simulink model "LaneMerge"  (Simulink 8.2)
settings: Solver=ode1  StartTime=0.0  StopTime=Inf  FixedStep=0.001  RelTol=1e-3
PostLoadFcn:
  | , if any(exist('dsrtsu_mdlpostloadfcn', 'file') == [2, 3, 6]), try dsrtsu_mdlpostloadfcn('Execute', bdroot); catch fprintf('Error in PostLoadFcn (dsrtsu_mdlpostloadfcn) for model "%s":\n %s\n', bdroot, lasterr); end, end,
undefined symbols (not defined in the file): AccelCommandMode, command_mode, max_accel_m_s2, MergeStateEnum, override_enabled, speed_command_m_s, VehicleRoleEnum, wrench_effort_command
libraries: simulink x19, merge_activation_lib x5, dsrc_util_lib x4, dsrc_transmitter x3, carma_platform x3, srx_platform x3, merge_control_lib x2, gap_controller_lib x2, rtitttasklib x2, command_handler_lib x1, vehicle_role_lib x1, simulink_utils_lib x1
settings Model: DSRTSU_INTERNAL_RTI_VER=450  DSRTSU_INTERNAL_RTI_TYPE=rti1401  DSRTSU_INTERNAL_RTIFPGA=40  Creator=rushk1  LastModifiedBy=rushk1  BufferReuse=off
settings DataIOCC: SignalLoggingSaveFormat=Dataset
settings OptimizationCC: BlockReduction=off  OptimizeBlockIOStorage=off  BufferReuse=off  ExpressionFolding=off  ExpressionDepthLimit=128  LocalBlockOutputs=off
settings DebuggingCC: FcnCallInpInsideContextMsg=EnableAllAsError  StateNameClashWarn=none
settings HardwareCC: ProdIntDivRoundTo=Zero  ProdEndianess=BigEndian  ProdHWDeviceType=Generic->Custom  TargetHWDeviceType=Generic->Custom
settings RTWCC: SystemTargetFile=rti1401.tlc  MakeCommand=make_rti  TemplateMakefile=rti1401.tmf  Description=dSPACE DS1401 Hardware Platform  ProcessScript=rti1401_make_rtw_hook  CustomSource=command_accel_encode.c
settings STFCustomTargetCC: CodeReplacementLibrary=ANSI_C  ParMdlRefBuildCompliant=on  GeneratePreprocessorConditionals=Disable all  SystemTargetFile=rti1401.tlc
settings GRTTargetCC: CompOptLevelCompliant=off  ConcurrentExecutionCompliant=off  MatFileLogging=off  ExtModeMexFile=noextcomm
settings CustomProperty: DataType=RTWOptions_EnumType_C__Program Files_dSPACE RCPHIL 2014-B_MATLAB_RTI_RTI1401_TLC_rti1401_1InitialSimState  Value=RUN
settings EnumStrPairs: String=RUN

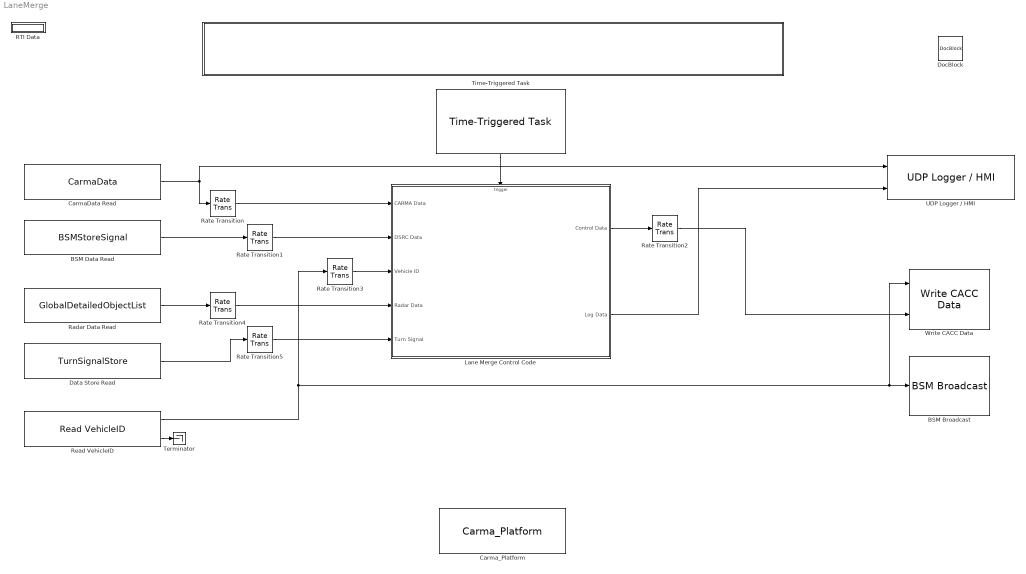
== system LaneMerge ==
  " " : Subsystem
      mask Display: disp('Lane Merge Control Software\nTOPR 20\n2015')
  BSM Broadcast : dsrc_transmitter/BSM Broadcast
  BSM Data Read : DataStoreRead  DataStoreName=BSMStoreSignal
  CarmaData Read : DataStoreRead  DataStoreName=CarmaData
  "Carma_Platform " : carma_platform/Carma_Platform 
  Data Store Read : DataStoreRead  DataStoreName=TurnSignalStore
  DocBlock : simulink/Model-Wide Utilities/DocBlock  DocumentType=Text
  Lane Merge Control Code : Subsystem
  RTI Data : Subsystem  Tag=struct('RTIDataServer',struct('RTIDataServerVs','2','RTIModelDescription','struct(''main'',''LaneMerge'',''sub'','''',''isMp'',0)'))  LoadFcn="if exist('rtidc'), try,  rtidc('DataHostBlockClbLoad', gcbh); catch, disp(['Warning: ''LoadFcn'' for RTI Data block failed: ' lasterr]); end, end,"  mask(RTI_DATA_HOST){}
      mask help:
      | RTI Data Block.
      | This block is used by RTI to store internal model-dependent data.
      | Please keep this block on the root level of the model. Deleting this block will result in data loss.
      |
      | NEVER DELETE OR COPY THIS BLOCK!
      settings: CopyFcn="if exist('rtidc'), try,  rtidc('DataHostBlockClbCopy', gcbh); catch, disp(['Warning: ''CopyFcn'' for RTI Data block failed: ' lasterr]); end, end,"  DeleteFcn="if exist('rtidc'), try,  rtidc('DataHostBlockClbDelete', gcbh); catch, disp(['Warning: ''DeleteFcn'' for RTI Data block failed: ' lasterr]); end, end,"  ModelCloseFcn="if exist('rtidc'), try,  rtidc('DataHostBlockClbModelClose', gcbh); catch, disp(['Warning: ''ModelCloseFcn'' for RTI Data block failed: ' lasterr]); end, end,"  PreSaveFcn="if exist('rtidc'), try,  rtidc('DataHostBlockClbPreSave', gcbh); catch, disp(['Warning: ''PreSaveFcn'' for RTI Data block failed: ' lasterr]); end, end,"  PostSaveFcn="if exist('rtidc'), try,  rtidc('DataHostBlockClbPostSave', gcbh); catch, disp(['Warning: ''PostSaveFcn'' for RTI Data block failed: ' lasterr]); end, end,"  NameChangeFcn="if exist('rtidc'), try,  rtidc('DataHostBlockClbNameChange', gcbh); catch, disp(['Warning: ''NameChangeFcn'' for RTI Data block failed: ' lasterr]); end, end,"
      mask Help:
      | RTI Data Block.
      | This block is used by RTI to store internal model-dependent data.
      | Please keep this block on the root level of the model. Deleting this block will result in data loss.
      | 
      | NEVER DELETE OR COPY THIS BLOCK!
      mask Display:
      | text(0.5, 0.5, 'RTI Data', 'HorizontalAlignment', 'center');
      | plot([1 0]);
  Radar Data Read : DataStoreRead  DataStoreName=GlobalDetailedObjectList
  Rate Transition{,1..5} (6 alike) : RateTransition  Deterministic=off
  Read VehicleID : srx_platform/Read VehicleID
  Terminator : Terminator
  Time-Triggered Task : rtitttasklib/Time-Triggered Task  TimeTriggerId=ALGO_EXEC  TLCFileName=rtitimetriggeredtask  DSProperties=struct('RTI',struct('Version',uint32(1),'BlockType',struct('isSLSource',uint8(1),'isSLSink',uint8(0),'isHWSource',uint8(0),'isHWSink',uint8(0),'isSetup',uint8(0),'isInline',uint8(1),'isNonInline',uint8(0),'isInterrupt',uint8(0),'isChannelwise',uint8(0)),'IOBoardType','RTITIMETRIGGER','UnitType','TIMETRIGGERED','Identifier','TASK','DialogType','SL','BlockSet','NONE','SlaveProcessor','NONE'))  RTIBlockInterface=struct('OutputPortsActive',1,'OutputPortsWidth',int32(1),'FunctionCall',uint32(0),'OutputPortsName',{{[' ']}},'InitLevel',3,'BlockDisplay',{{['Time-Triggered Task\nID: ''''ALGO_EXEC'''''],'center'}},'IconTransparency','off','BlockName',struct('Token',{{['Time-Triggered Task']}}),'MaskDescription',['Specifies a time-triggered task. The task trigger times are set by the assigned Time-Trigger Set block.' char(10) '' char(10) 'This block can only be used together with the Time-Trigger Set block.'])  RTIBlockParameters=struct('TimeTriggerId',{{'ALGO_EXEC','OFF',[]}},'TLCFileName',{{'rtitimetriggeredtask','OFF',[]}})  RTISFcnParameters=struct('TLCFileName','char')  RTIBlockParaDefault=struct('TimeTriggerId','TT_ID','TLCFileName','rtitimetriggeredtask')
  UDP Logger / HMI : carma_platform/UDP Logger // HMI  Value=0.05
  Write CACC Data : dsrc_transmitter/Write CACC Data
  wires:
  BSM Data Read/1 -> Rate Transition1/1
  CarmaData Read/1 -> Rate Transition/1, UDP Logger / HMI/1
  Rate Transition1/1 -> Lane Merge Control Code/2(DSRC Data)
  Lane Merge Control Code/2(Log Data) -> UDP Logger / HMI/2
  Lane Merge Control Code/1(Control Data) -> Rate Transition2/1
  Read VehicleID/2 -> Terminator/1
  Read VehicleID/1 -> Write CACC Data/1, BSM Broadcast/1, Rate Transition3/1
  Rate Transition2/1 -> Write CACC Data/2
  Time-Triggered Task/1 -> Lane Merge Control Code/Trigger
  Rate Transition3/1 -> Lane Merge Control Code/3(Vehicle ID)
  Rate Transition/1 -> Lane Merge Control Code/1(CARMA Data)
  Radar Data Read/1 -> Rate Transition4/1
  Rate Transition4/1 -> Lane Merge Control Code/4(Radar Data)
  Data Store Read/1 -> Rate Transition5/1
  Rate Transition5/1 -> Lane Merge Control Code/5(Turn Signal)

== system LaneMerge/  ==

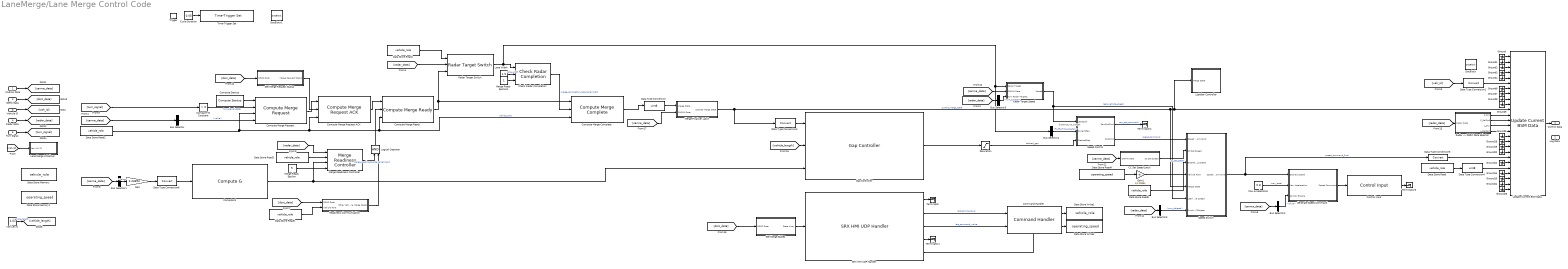
== system LaneMerge/Lane Merge Control Code ==
  note: distance_to_target
  CARMA Data : Inport
  DSRC Data : Inport  Port=2
  Vehicle ID : Inport  Port=3
  Radar Data : Inport  Port=4  OutDataTypeStr=Bus: DetailedObjectList
  Turn Signal : Inport  Port=5
  Trigger : TriggerPort  TriggerType=function-call  PortDimensions=1
  Bus Selector : BusSelector  OutputSignals=acc_status.value
  Bus Selector1 : BusSelector  OutputSignals=speed_m_s.value
  Bus Selector2 : BusSelector  OutputSignals=acc_status.value
  Bus Selector3 : BusSelector  OutputSignals=num_objects
  Bus Selector4 : BusSelector  OutputSignals=FwdFusTrkALongPos
  Bus Selector5 : BusSelector  OutputSignals=num_objects
  CC Set Speed Latch : Subsystem  TreatAsAtomicUnit=on
  Check Radar Completion : merge_control_lib/Check Radar Completion
  Command Handler : command_handler_lib/Command Handler
  Compare To Constant : simulink/Logic and Bit Operations/Compare To Constant  relop=>  const=0  OutDataTypeStr=boolean
  Compute G : gap_controller_lib/Compute G
  Compute Merge Complete : merge_activation_lib/Compute Merge Complete
  Compute Merge Ready : merge_activation_lib/Compute Merge Ready
  Compute Merge Request : merge_activation_lib/Compute Merge Request
  Compute Merge Request ACK : merge_activation_lib/Compute Merge Request ACK
  Compute Startup : merge_activation_lib/Compute Startup
  Control Input : carma_platform/Control Input
  Cycle Duration : Constant  Value=0.05
  Data Store Memory : DataStoreMemory  DataStoreName=vehicle_role  ReadBeforeWriteMsg=warning  WriteAfterWriteMsg=warning  WriteAfterReadMsg=warning  InitialValue=VehicleRoleEnum.ERROR
  Data Store Memory1 : DataStoreMemory  DataStoreName=operating_speed  ReadBeforeWriteMsg=warning  WriteAfterWriteMsg=warning  WriteAfterReadMsg=warning  InitialValue=25
  Data Store Read{,1..3,5..6} (6 alike) : DataStoreRead  DataStoreName=vehicle_role
  Data Store Read4 : DataStoreRead  DataStoreName=operating_speed
  Data Store Write1 : DataStoreWrite  DataStoreName=vehicle_role
  Data Store Write2 : DataStoreWrite  DataStoreName=operating_speed
  Data Type Conversion : DataTypeConversion  OutDataTypeStr=uint8
  Data Type Conversion{1,3,5..6} (4 alike) : DataTypeConversion
  Data Type Conversion4 : DataTypeConversion  OutDataTypeStr=uint8
  DocBlock : simulink/Model-Wide Utilities/DocBlock  DocumentType=Text
  DocBlock1 : simulink/Model-Wide Utilities/DocBlock  DocumentType=Text
      content=|
      | Lane Merge Control Code
      | ===========================================================================
      | This subystem contains all of the algorithm logic for the Lane Merge
      | application.
      |
      | This logic is executed at a 20hz timestep with hard real time deadlines.
      | During each iteration the following steps are performed:
      |
      | 1) Receive inputs from the platform. The latest data is gathered from the
      | relevant storage buffers (being updated by other code on independent time
      | basis) and used to perform new computations.
      | 2) Recompute state. The state of the vehicle (as defined in
      | MergeStateEnum.m) is recomputed every timestep with the newly available
      | information. This ensures that all conditions are still met and handles
      | state changes and transitions in a consistent and reliable fashion.
      | 3) Compute desired gap. The desired gap to radar target is computed based
      | on current speed and merge state.
      | 4) Regulate gap. The speed controller uses a PID to minimize gap error by
      | speeding up or slowing down the vehicle relative to the radar target.
      | 5) Broadcast data. The new state, speed command, and other data is written
      | into the appropriate DSRC buffers and broadcasted.
  Gain : Gain  Gain=2.23694  OutDataTypeStr=single
  Gain1 : Gain  Gain=1/2.23694
  Gap Controller : gap_controller_lib/Gap Controller
  Generate Speed Command : Subsystem
  Get Merge Request Status : Subsystem
  Get Merge States : Subsystem
  Ground{,1..9,14..15,18..20,22,24..25} (18 alike) : Ground
  Lane Merge Initializer : Subsystem
  Lane Width : Constant  Value=1.5
  Lightbar Controller : Subsystem
  Logical Operator : Logic  IconShape=distinctive  AllPortsSameDT=off  OutDataTypeStr=boolean
  Max Acceleration : Constant  Value=0.8
  Merge Finalizer Latch : Subsystem
  Merge Readiness Controller : merge_control_lib/Merge Readiness Controller
  Merge Ready Epsilon : Constant  Value=5
  Merge Ready Epsilon1 : Constant
  "Radar -> DSRC Data Selector" : Subsystem
  Radar Target Speed : Subsystem
  Radar Target Switch : radar_switch_lib/Radar Target Switch
  Readiness Communication : Subsystem
  SRX HMI UDP Handler : hmi_udp_lib/SRX HMI UDP Handler
  Saturation : Saturate  UpperLimit=70  LowerLimit=4.83
  Speed Control : Subsystem
  Speed Switch : Subsystem
  Terminator{,1..3} (4 alike) : Terminator
  Time-Trigger Set : rtitttasklib/Time-Trigger Set  TimeTriggerId=ALGO_EXEC  SampleTime=-1  RegisterAtSimulationStart=on  TLCFileName=rtitimetriggerset  DSProperties=struct('RTI',struct('Version',uint32(1),'BlockType',struct('isSLSource',uint8(1),'isSLSink',uint8(0),'isHWSource',uint8(0),'isHWSink',uint8(0),'isSetup',uint8(0),'isInline',uint8(1),'isNonInline',uint8(0),'isInterrupt',uint8(0),'isChannelwise',uint8(0)),'IOBoardType','RTITIMETRIGGER','UnitType','TIMETRIGGERED','Identifier','SET','DialogType','SL','BlockSet','NONE','SlaveProcessor','NONE'))  RTIBlockInterface=struct('InputPortsActive',1,'InputPortsWidth',{{'DYNAMICALLY_SIZED'}},'InputPortsDataType',{{'SS_DOUBLE'}},'InputPortsName',{{['Trigger delay']}},'InitLevel',3,'BlockDisplay',{{['Time-Trigger Set\nID: ''''ALGO_EXEC'''''],'center'}},'IconTransparency','on','BlockName',struct('Token',{{['Time-Trigger Set']}}),'MaskDescription',['When this block is evaluated it sets the task trigger times for the assigned time-triggered task.' char(10) '' char(10) 'This block can only be used together with the Time-Triggered Task block.'],'SampleTime',{{-1}})  RTIBlockParameters=struct('TimeTriggerId',{{'ALGO_EXEC','OFF',[]}},'SampleTime',{{-1,'OFF',[]}},'RegisterAtSimulationStart',{{logical(1),'OFF',[]}},'TLCFileName',{{'rtitimetriggerset','OFF',[]}})  RTISFcnParameters=struct('TimeTriggerId','char','SampleTime','double','TLCFileName','char','RegisterAtSimulationStart','double')  RTIBlockParaDefault=struct('TimeTriggerId','TT_ID','SampleTime',-1,'RegisterAtSimulationStart',0,'TLCFileName','rtitimetriggerset')
  Update Current BSM Data : dsrc_transmitter/Update Current BSM Data
  Veh Len m : Constant  Value=4.83
  Control Data : Outport
  Log Data : Outport  Port=2
  wires:
  Vehicle ID/1 -> [veh_id]
  Cycle Duration/1 -> Time-Trigger Set/1
  Update Current BSM Data/1 -> Control Data/1
  Ground/1 -> Update Current BSM Data/1
  Ground1/1 -> Update Current BSM Data/2
  Ground2/1 -> Update Current BSM Data/3
  Ground3/1 -> Update Current BSM Data/4
  Ground4/1 -> Update Current BSM Data/5
  Ground9/1 -> Update Current BSM Data/10
  Ground7/1 -> Update Current BSM Data/8
  Ground8/1 -> Update Current BSM Data/9
  Ground6/1 -> Update Current BSM Data/7
  Ground22/1 -> Update Current BSM Data/21
  Ground15/1 -> Update Current BSM Data/24
  Ground19/1 -> Update Current BSM Data/18
  Ground18/1 -> Update Current BSM Data/17
  Ground14/1 -> Update Current BSM Data/23
  Data Store Read/1 -> Data Type Conversion4/1
  Ground20/1 -> Update Current BSM Data/19
  Ground24/1 -> Update Current BSM Data/25
  Ground25/1 -> Update Current BSM Data/26
  Radar Data/1 -> [radar_data]
  CARMA Data/1 -> [carma_data]
  Merge Finalizer Latch/1(Latched Merge State) -> Data Type Conversion3/1, Speed Switch/5(Merge State), Lightbar Controller/1(Merge State), Update Current BSM Data/11  "current_merge_state"
  Data Type Conversion1/1 -> Update Current BSM Data/6
  Lane Width/1 -> Check Radar Completion/2  "lane_width"
  [veh_id] -> Lane Merge Initializer/1(Veh HW ID)
  [carma_data] -> Bus Selector/1
  DSRC Data/1 -> [dsrc_data]
  [radar_data] -> Merge Readiness Controller/1
  Data Store Read3/1 -> Merge Readiness Controller/2
  [veh_id] -> Data Type Conversion1/1
  Data Type Conversion3/1 -> Gap Controller/1
  Data Type Conversion4/1 -> Update Current BSM Data/22
  SRX HMI UDP Handler/2 -> Command Handler/1  "last_command_id"
  SRX HMI UDP Handler/3 -> Command Handler/2  "last_command_value"
  Command Handler/1 -> Data Store Write1/1
  Command Handler/2 -> Data Store Write2/1
  SRX HMI UDP Handler/5 -> Command Handler/Enable
  SRX HMI UDP Handler/1 -> Terminator/1
  [radar_data] -> Radar Target Switch/2
  Radar Target Switch/1 -> Check Radar Completion/1, Bus Selector4/1, Radar Target Speed/1(Radar Target)
  Speed Control/2(SpdCmd) -> Speed Switch/1(Speed Controller Command)  "speed_command"
  Speed Control/1(RawSpdCmd) -> Terminator2/1  "raw_spd_command"
  Control Input/1 -> Terminator3/1
  Speed Switch/1(Speed Command) -> Data Type Conversion5/1, Generate Speed Command/1(Desired Speed)  "speed_command_final"
  Data Store Read4/1 -> Gain1/1
  Generate Speed Command/1(Speed Command) -> Control Input/1
  Bus Selector2/1 -> Generate Speed Command/3(Control Enable)  "<value>"
  [carma_data] -> Bus Selector2/1
  Max Acceleration/1 -> Generate Speed Command/2(Max Acceleration)  "max_accel"
  Get Merge States/1(State Array) -> SRX HMI UDP Handler/1
  Compute G/1 -> Merge Readiness Controller/3, Gap Controller/3
  Radar Target Speed/1(Speed) -> Speed Switch/6(Lead Vehicle Speed), Speed Control/1(LeadSpd)  "lead_vehicle_speed"
  Data Store Read2/1 -> Compute Merge Request/3, Compute Merge Request ACK/3, Compute Merge Complete/3, Compute Merge Ready/3  "vehicle_role"
  Compute Merge Request/1 -> Compute Merge Request ACK/1
  [turn_signal] -> Compare To Constant/1
  Compute Startup/1 -> Compute Merge Request/1
  Merge Readiness Controller/1 -> Logical Operator/1  "merge_readiness_radar_alignment"
  Compute Merge Ready/1 -> Radar Target Switch/3, Compute Merge Complete/1
  Check Radar Completion/1 -> Compute Merge Complete/2  "merge_completion_radar_alignment"
  Compute Merge Request ACK/1 -> Compute Merge Ready/1
  Bus Selector/1 -> Compute Merge Request/4  "<value>"
  Turn Signal/1 -> [turn_signal]
  Compare To Constant/1 -> Compute Merge Request/2  "turn_signal_state"
  Data Store Read5/1 -> Speed Switch/4(Vehicle Role)
  CC Set Speed Latch/1(CC Set Speed) -> Speed Switch/2(CC Set Speed)  "cc_set_speed"
  [carma_data] -> CC Set Speed Latch/1(CARMA Data)
  Ground5/1 -> Update Current BSM Data/16
  Get Merge Request Status/1(Merge Request Status) -> Compute Merge Request ACK/2
  [dsrc_data] -> Get Merge Request Status/1(DSRC Data)
  [radar_data] -> "Radar -> DSRC Data Selector"/1(Radar Data)
  "Radar -> DSRC Data Selector"/1(P_Dis) -> Update Current BSM Data/12
  "Radar -> DSRC Data Selector"/2(P_RelSpd) -> Update Current BSM Data/13
  "Radar -> DSRC Data Selector"/3(L_Dis) -> Update Current BSM Data/14
  "Radar -> DSRC Data Selector"/4(L_RelSpd) -> Update Current BSM Data/15
  Data Type Conversion5/1 -> Update Current BSM Data/20
  Gain1/1 -> Speed Switch/3(Operating Speed)
  [carma_data] -> Radar Target Speed/2(CARMA Data)
  Saturation/1 -> Speed Control/3(DesiredGap)  "desired_gap"
  Veh Len m/1 -> [vehicle_length]  "vehicle_length"
  [vehicle_length] -> Gap Controller/2
  Data Store Read1/1 -> Radar Target Switch/1
  [radar_data] -> Bus Selector3/1
  Bus Selector3/1 -> Radar Target Speed/3(Num Radar Targets)  "<num_objects>"
  Bus Selector4/1 -> Speed Control/2(CurrentGap)  "<FwdFusTrkALongPos>"
  Data Store Read6/1 -> Readiness Communication/2(Vehicle Role)
  [dsrc_data] -> Readiness Communication/1(DSRC Data)
  Readiness Communication/1(Other Vehicle Merge Ready) -> Logical Operator/2
  Logical Operator/1 -> Compute Merge Ready/2
  [dsrc_data] -> Get Merge States/1(DSRC Data)
  [carma_data] -> Bus Selector1/1
  Bus Selector1/1 -> Gain/1  "<value>"
  Gain/1 -> Data Type Conversion6/1
  Data Type Conversion6/1 -> Compute G/1
  SRX HMI UDP Handler/4 -> Terminator1/1
  Merge Ready Epsilon/1 -> Merge Readiness Controller/4
  Merge Ready Epsilon1/1 -> Check Radar Completion/3
  [radar_data] -> Bus Selector5/1
  Bus Selector5/1 -> Speed Switch/7(Number of Objects)  "<num_objects>"
  Compute Merge Complete/1 -> Data Type Conversion/1
  [carma_data] -> Merge Finalizer Latch/2(CARMA Data)
  Data Type Conversion/1 -> Merge Finalizer Latch/1(Merge State)
  Gap Controller/1 -> Saturation/1

== system LaneMerge/RTI Data ==
  RTI Data Store : Subsystem  Tag="struct('private',struct('version',struct('dsVer',uint32(2),'dsVerCreation',uint32(2),'RTI',struct('ver','7.3','type','RTI1401')),'access',struct('type','Model','isPerm',1,'created',['07-Dec-2015 11:46:35'],'modified',['06-Jan-2016 14:59:22'],'location','')),'public',struct('main',struct('data',[]),'sub',struct('name',{{'LaneMerge'}},'data',{{struct('TH',struct('thTaskInfo',struct('taskType',{'TIMER','HWINT','TMRINT','SWINT','GLINT'},'tasksNumOf',{1,1,3,0,0},'srcIds',{{'TIMERA'},{'BB_BYP_ETHT1M0I0S0'},{'INTERVALA1','INTERVALA2','INTERVALA3'},{},{}},'taskNames',{{['Timer Task 1']},{['rti_ethernet_interface_name Interrupt [RX/TX]']},{['BSM Broadcast Task'],['Time-Triggered Task'],['test trigger']},{},{}})),'th_tc',struct('dataType',{'TASK','TASK','TASK','TASK','TASK'},'taskGroupId',{'','','','',''},'taskGroupList',{{},{},{},{},{}},'taskSchedulingPolicy',{'FCFS','FCFS','FCFS','FCFS','FCFS'},'taskType',{'TIMER','HWINT','TMRINT','TMRINT','TMRINT'},'blkh',{-1,['LaneMerge/Carma_Platform' char(10) '/SRX Platform Initializer/SRX UDP Initializer/ETHERNET_UDP_SETUP_BL1/Common Hardware' char(10) 'Interrupt Interface'],['LaneMerge/BSM Broadcast/BSM Broadcast Task/Common Timer' char(10) 'Interrupt Interface'],['LaneMerge/Time-Triggered Task/Common Timer' char(10) 'Interrupt Interface'],['LaneMerge/UDP Logger // HMI/test trigger/Common Timer' char(10) 'Interrupt Interface']},'srcId',{'TIMERA','BB_BYP_ETHT1M0I0S0','INTERVALA1','INTERVALA2','INTERVALA3'},'srcSgnName',{['Timer A interrupt'],['BB_BYP_ETH Type 1 Module 1 HW-Int 0 Interrupt 0'],['Interval Timer A'],['Interval Timer A'],['Interval Timer A']},'srcCpuName',{'','','','',''},'taskName',{['Timer Task 1  [0.001] s'],['rti_ethernet_interface_name Interrupt [RX/TX]'],['BSM Broadcast Task'],['Time-Triggered Task'],['test trigger']},'taskNameDisplayExt',{'','','','',''},'smplTime',{0.001,0,0,0,0},'smplTimeOffs',{0,0,0,0,0},'hasFixedPriority',{0,0,0,0,0},'priority',{3,2,4,1,5},'hasFixedOvc',{0,0,0,0,0},'ovcType',{1,1,1,1,1},'ovcMax',{1,1,1,1,1}),'tc_th',struct('dataType',{'TASK','TASK','TASK','TASK','TASK'},'taskGroupId',{'','','','',''},'taskGroupList',{{},{},{},{},{}},'taskSchedulingPolicy',{'FCFS','FCFS','FCFS','FCFS','FCFS'},'taskType',{'TIMER','HWINT','TMRINT','TMRINT','TMRINT'},'blkh',{-1,['LaneMerge/Carma_Platform' char(10) '/SRX Platform Initializer/SRX UDP Initializer/ETHERNET_UDP_SETUP_BL1/Common Hardware' char(10) 'Interrupt Interface'],['LaneMerge/BSM Broadcast/BSM Broadcast Task/Common Timer' char(10) 'Interrupt Interface'],['LaneMerge/Time-Triggered Task/Common Timer' char(10) 'Interrupt Interface'],['LaneMerge/UDP Logger // HMI/test trigger/Common Timer' char(10) 'Interrupt Interface']},'srcId',{'TIMERA','BB_BYP_ETHT1M0I0S0','INTERVALA1','INTERVALA2','INTERVALA3'},'srcSgnName',{['Timer A interrupt'],['BB_BYP_ETH Type 1 Module 1 HW-Int 0 Interrupt 0'],['Interval Timer A'],['Interval Timer A'],['Interval Timer A']},'srcCpuName',{'','','','',''},'taskName',{['Timer Task 1  [0.001] s'],['rti_ethernet_interface_name Interrupt [RX/TX]'],['BSM Broadcast Task'],['Time-Triggered Task'],['test trigger']},'taskNameDisplayExt',{'','','','',''},'smplTime',{0.001,0,0,0,0},'smplTimeOffs',{0,0,0,0,0},'hasFixedPriority',{0,0,0,0,0},'priority',{3,2,4,1,5},'hasFixedOvc',{0,0,0,0,0},'ovcType',{1,1,1,1,1},'ovcMax',{1,1,1,1,1}))}})))"  mask(RTI_DATA_STORE){}
      mask help:
      | RTI Data Store Block. This block is used by RTI to store internal model dependent data. Deleting this block will result in data loss.
      |
      | NEVER DELETE, COPY, OR MODIFY THIS BLOCK!
      mask Help:
      | RTI Data Store Block. This block is used by RTI to store internal model dependent data. Deleting this block will result in data loss.
      | 
      | NEVER DELETE, COPY, OR MODIFY THIS BLOCK!
      mask Display: text(0.5, 0.5, ' ', 'HorizontalAlignment', 'center');

== system LaneMerge/Lane Merge Control Code/CC Set Speed Latch ==
  CARMA Data : Inport  OutDataTypeStr=Bus: GlobalStoreBus
  Bus Selector : BusSelector  OutputSignals=acc_status.value,speed_m_s.value
  Data Store Read : DataStoreRead  DataStoreName=set_speed
  Data Type Conversion : DataTypeConversion
  DocBlock : simulink/Model-Wide Utilities/DocBlock  DocumentType=Text
  Latch Set : Subsystem  TreatAsAtomicUnit=on
  Set Speed Latch : DataStoreMemory  DataStoreName=set_speed  ReadBeforeWriteMsg=warning  WriteAfterWriteMsg=warning  WriteAfterReadMsg=warning  InitialValue=25
  CC Set Speed : Outport
  wires:
  CARMA Data/1 -> Bus Selector/1
  Bus Selector/1 -> Latch Set/Trigger  "<value>"
  Bus Selector/2 -> Latch Set/1(In1)  "<value>"
  Data Store Read/1 -> Data Type Conversion/1
  Data Type Conversion/1 -> CC Set Speed/1

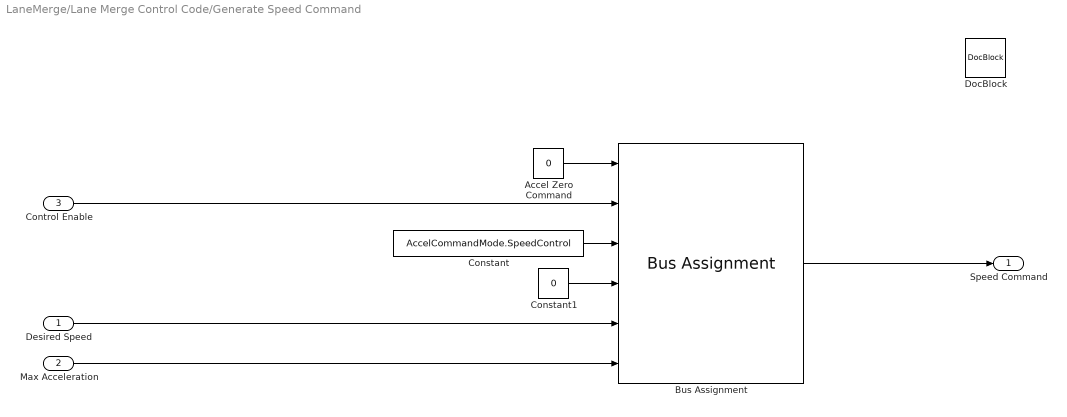
== system LaneMerge/Lane Merge Control Code/Generate Speed Command ==
  Desired Speed : Inport
  Max Acceleration : Inport  Port=2
  Control Enable : Inport  Port=3
  Accel Zero Command : Constant  Value=0  OutDataTypeStr=Bus: AccelCommandBus
  Bus Assignment : BusAssignment  AssignedSignals=override_enabled,command_mode,wrench_effort_command,speed_command_m_s,max_accel_m_s2
  Constant : Constant  Value=AccelCommandMode.SpeedControl  OutDataTypeStr=Enum: AccelCommandMode
  Constant1 : Constant  Value=0
  DocBlock : simulink/Model-Wide Utilities/DocBlock  DocumentType=Text
  Speed Command : Outport
  wires:
  Control Enable/1 -> Bus Assignment/2
  Constant1/1 -> Bus Assignment/4
  Desired Speed/1 -> Bus Assignment/5
  Max Acceleration/1 -> Bus Assignment/6
  Accel Zero Command/1 -> Bus Assignment/1
  Bus Assignment/1 -> Speed Command/1
  Constant/1 -> Bus Assignment/3

== system LaneMerge/Lane Merge Control Code/Get Merge Request Status ==
  DSRC Data : Inport  OutDataTypeStr=Bus: BSMStoreBus
  Bus Selector : BusSelector  OutputSignals=vehManID
  Compare To Constant : simulink/Logic and Bit Operations/Compare To Constant  relop=>=  const=1  OutDataTypeStr=boolean
  Constant : Constant  Value=VehicleRoleEnum.MERGE
  Data Type Conversion : DataTypeConversion
  Get BSM for Role : dsrc_util_lib/Get BSM for Role
  Merge Request Status : Outport
  wires:
  DSRC Data/1 -> Get BSM for Role/1
  Constant/1 -> Get BSM for Role/2
  Get BSM for Role/1 -> Bus Selector/1
  Bus Selector/1 -> Data Type Conversion/1  "<vehManID>"
  Compare To Constant/1 -> Merge Request Status/1
  Data Type Conversion/1 -> Compare To Constant/1

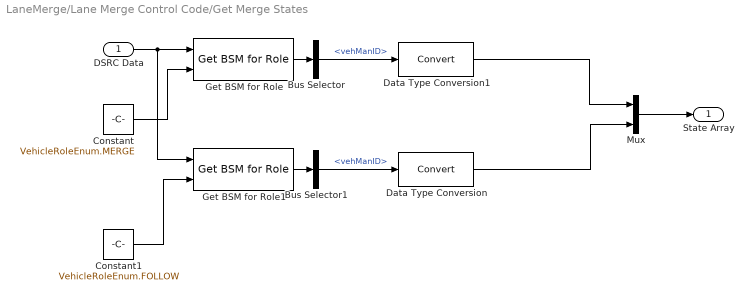
== system LaneMerge/Lane Merge Control Code/Get Merge States ==
  DSRC Data : Inport  OutDataTypeStr=Bus: BSMStoreBus
  Bus Selector : BusSelector  OutputSignals=vehManID
  Bus Selector1 : BusSelector  OutputSignals=vehManID
  Constant : Constant  Value=VehicleRoleEnum.MERGE
  Constant1 : Constant  Value=VehicleRoleEnum.FOLLOW
  Data Type Conversion : DataTypeConversion
  Data Type Conversion1 : DataTypeConversion
  Get BSM for Role : dsrc_util_lib/Get BSM for Role
  Get BSM for Role1 : dsrc_util_lib/Get BSM for Role
  Mux : Mux  Inputs=2
  State Array : Outport
  wires:
  DSRC Data/1 -> Get BSM for Role/1, Get BSM for Role1/1
  Constant/1 -> Get BSM for Role/2
  Constant1/1 -> Get BSM for Role1/2
  Get BSM for Role/1 -> Bus Selector/1
  Get BSM for Role1/1 -> Bus Selector1/1
  Bus Selector/1 -> Data Type Conversion1/1  "<vehManID>"
  Bus Selector1/1 -> Data Type Conversion/1  "<vehManID>"
  Mux/1 -> State Array/1
  Data Type Conversion/1 -> Mux/2
  Data Type Conversion1/1 -> Mux/1

== system LaneMerge/Lane Merge Control Code/Lane Merge Initializer ==
  Veh HW ID : Inport
  Data Store Read2 : DataStoreRead  DataStoreName=vehicle_role
  Data Store Write : DataStoreWrite  DataStoreName=vehicle_role
  DocBlock : simulink/Model-Wide Utilities/DocBlock  DocumentType=Text
  Vehicle Role Determinator : vehicle_role_lib/Vehicle Role Determinator
  wires:
  Vehicle Role Determinator/1 -> Data Store Write/1
  Veh HW ID/1 -> Vehicle Role Determinator/1
  Data Store Read2/1 -> Vehicle Role Determinator/2

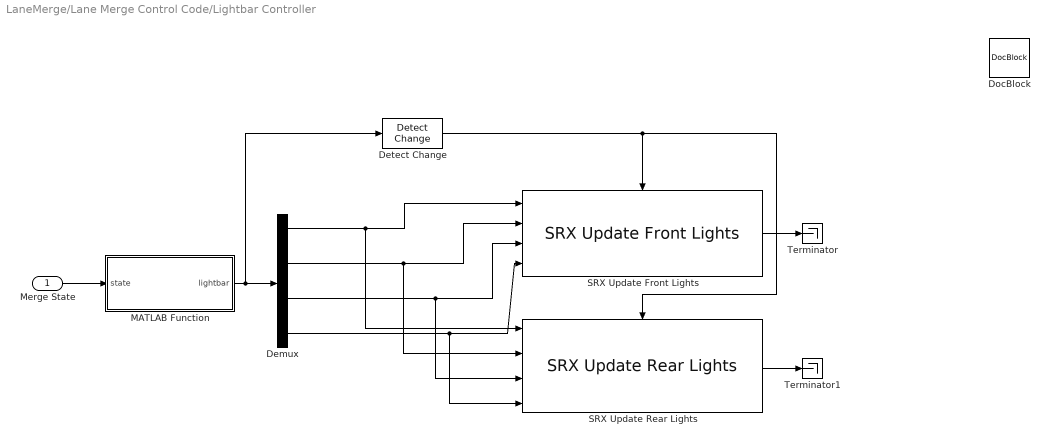
== system LaneMerge/Lane Merge Control Code/Lightbar Controller ==
  Merge State : Inport
  Demux : Demux
  Detect Change : simulink/Logic and Bit Operations/Detect Change  vinit=0  InputProcessing=Inherited  OutDataTypeStr=boolean
  DocBlock : simulink/Model-Wide Utilities/DocBlock  DocumentType=Text
      content=|
      | This block is responsible for controlling the state of the vehicle's
      | lightbar.
      |
      | The lightbar state is dependant on the vehicle's merge state. Merge request
      | triggers the right side of the lightbar to flash. Merge request ack
      | triggers the left side of the bar to flash. Merge ready causes both sides
      | of the lightbar to flash. Once merge completion is attained the green light
      | in the center of light bar will light up solid.
  MATLAB Function : MATLAB Function  TreatAsAtomicUnit=on
  SRX Update Front Lights : srx_platform/SRX Update Front Lights
  SRX Update Rear Lights : srx_platform/SRX Update Rear Lights
  Terminator : Terminator
  Terminator1 : Terminator
  wires:
  Demux/1 -> SRX Update Rear Lights/1, SRX Update Front Lights/1
  Demux/2 -> SRX Update Rear Lights/2, SRX Update Front Lights/2
  Demux/3 -> SRX Update Rear Lights/3, SRX Update Front Lights/3
  Demux/4 -> SRX Update Rear Lights/4, SRX Update Front Lights/4
  MATLAB Function/1(lightbar) -> Detect Change/1, Demux/1
  Merge State/1 -> MATLAB Function/1(state)
  Detect Change/1 -> SRX Update Front Lights/Enable, SRX Update Rear Lights/Enable
  SRX Update Front Lights/1 -> Terminator/1
  SRX Update Rear Lights/1 -> Terminator1/1

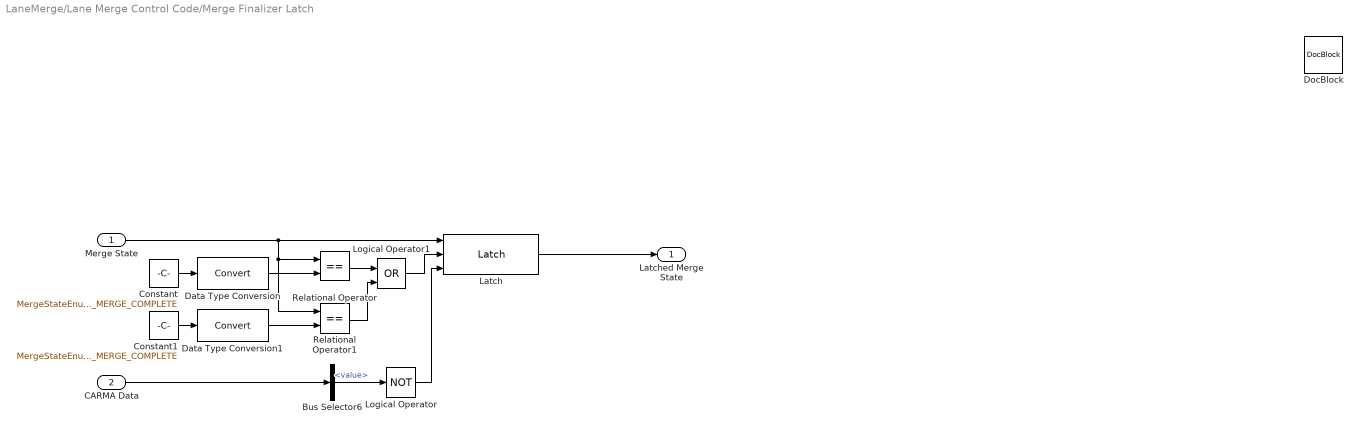
== system LaneMerge/Lane Merge Control Code/Merge Finalizer Latch ==
  Merge State : Inport
  CARMA Data : Inport  Port=2
  Bus Selector6 : BusSelector  OutputSignals=acc_status.value
  Constant : Constant  Value=MergeStateEnum.F_MERGE_COMPLETE
  Constant1 : Constant  Value=MergeStateEnum.M_MERGE_COMPLETE
  Data Type Conversion : DataTypeConversion
  Data Type Conversion1 : DataTypeConversion
  DocBlock : simulink/Model-Wide Utilities/DocBlock  DocumentType=Text
      content=|
      | This block is responsible for latching the merge completion state.
      |
      | Once F_MERGE_COMPLETE or M_MERGE_COMPLETE has been held for 20 timesteps
      | (1 second real time) it is held until the ACC system is disabled.
  Latch : simulink_utils_lib/Latch  timestep_threshold=20
  Logical Operator : Logic  Operator=NOT  IconShape=distinctive  AllPortsSameDT=off  OutDataTypeStr=boolean
  Logical Operator1 : Logic  Operator=OR  IconShape=distinctive  AllPortsSameDT=off  OutDataTypeStr=boolean
  Relational Operator : RelationalOperator  Operator===  OutDataTypeStr=boolean
  Relational Operator1 : RelationalOperator  Operator===  OutDataTypeStr=boolean
  Latched Merge State : Outport
  wires:
  Relational Operator/1 -> Logical Operator1/1
  Constant/1 -> Data Type Conversion/1
  Merge State/1 -> Relational Operator1/1, Relational Operator/1, Latch/1
  Relational Operator1/1 -> Logical Operator1/2
  CARMA Data/1 -> Bus Selector6/1
  Logical Operator1/1 -> Latch/2
  Constant1/1 -> Data Type Conversion1/1
  Latch/1 -> Latched Merge State/1
  Bus Selector6/1 -> Logical Operator/1  "<value>"
  Logical Operator/1 -> Latch/3
  Data Type Conversion/1 -> Relational Operator/2
  Data Type Conversion1/1 -> Relational Operator1/2

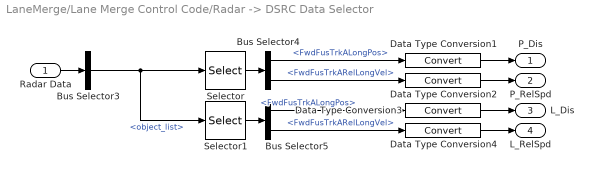
== system LaneMerge/Lane Merge Control Code/Radar -> DSRC Data Selector ==
  Radar Data : Inport
  Bus Selector3 : BusSelector  OutputSignals=object_list
  Bus Selector4 : BusSelector  OutputSignals=FwdFusTrkALongPos,FwdFusTrkARelLongVel
  Bus Selector5 : BusSelector  OutputSignals=FwdFusTrkALongPos,FwdFusTrkARelLongVel
  Data Type Conversion{1..4} (4 alike) : DataTypeConversion
  Selector : Selector  InputPortWidth=4  IndexOptions=Index vector (dialog)  Indices=[1]  OutputSizes=1
  Selector1 : Selector  InputPortWidth=4  IndexOptions=Index vector (dialog)  Indices=[2]  OutputSizes=1
  P_Dis : Outport
  P_RelSpd : Outport  Port=2
  L_Dis : Outport  Port=3
  L_RelSpd : Outport  Port=4
  wires:
  Bus Selector5/2 -> Data Type Conversion4/1  "<FwdFusTrkARelLongVel>"
  Bus Selector5/1 -> Data Type Conversion3/1  "<FwdFusTrkALongPos>"
  Radar Data/1 -> Bus Selector3/1
  Bus Selector4/2 -> Data Type Conversion2/1  "<FwdFusTrkARelLongVel>"
  Bus Selector3/1 -> Selector1/1, Selector/1  "<object_list>"
  Bus Selector4/1 -> Data Type Conversion1/1  "<FwdFusTrkALongPos>"
  Selector1/1 -> Bus Selector5/1
  Selector/1 -> Bus Selector4/1
  Data Type Conversion1/1 -> P_Dis/1
  Data Type Conversion2/1 -> P_RelSpd/1
  Data Type Conversion3/1 -> L_Dis/1
  Data Type Conversion4/1 -> L_RelSpd/1

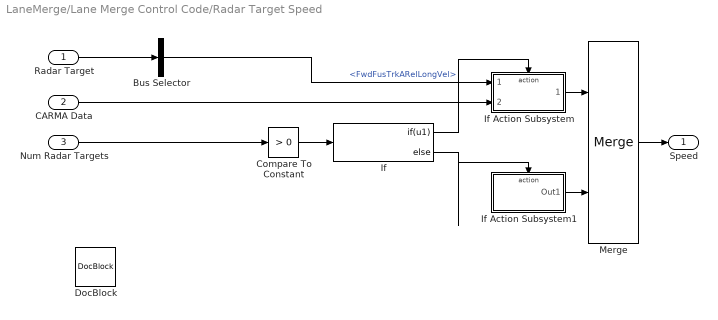
== system LaneMerge/Lane Merge Control Code/Radar Target Speed ==
  Radar Target : Inport  OutDataTypeStr=Bus: FusObjectTrackA
  CARMA Data : Inport  Port=2  OutDataTypeStr=Bus: GlobalStoreBus
  Num Radar Targets : Inport  Port=3
  Bus Selector : BusSelector  OutputSignals=FwdFusTrkARelLongVel
  Compare To Constant : simulink/Logic and Bit Operations/Compare To Constant  relop=>  const=0  OutDataTypeStr=boolean
  DocBlock : simulink/Model-Wide Utilities/DocBlock  DocumentType=Text
      content=|
      | This block computes the speed of the current radar target.
      |
      | The radar system returns a relative speed value so this block adds our
      | absolute speed to the relative speed of the radar target to get the radar
      | target's absolute speed.
      |
      | In the event of no radar objects we output zero (since the relative speed
      | is return as zero in this case by the radar system) to prevent runaway
      | acceleration events.
  If : If  IfExpression=u1
  If Action Subsystem : Subsystem  TreatAsAtomicUnit=on
  If Action Subsystem1 : Subsystem  TreatAsAtomicUnit=on
  Merge : Merge
  Speed : Outport
  wires:
  If/1 -> If Action Subsystem/Action
  If/2 -> If Action Subsystem1/Action
  If Action Subsystem/1(Lead Vehicle Speed) -> Merge/1
  If Action Subsystem1/1(Out1) -> Merge/2
  Merge/1 -> Speed/1
  Compare To Constant/1 -> If/1
  CARMA Data/1 -> If Action Subsystem/2(CARMA Data)
  Num Radar Targets/1 -> Compare To Constant/1
  Radar Target/1 -> Bus Selector/1
  Bus Selector/1 -> If Action Subsystem/1(Relative Velocity)  "<FwdFusTrkARelLongVel>"

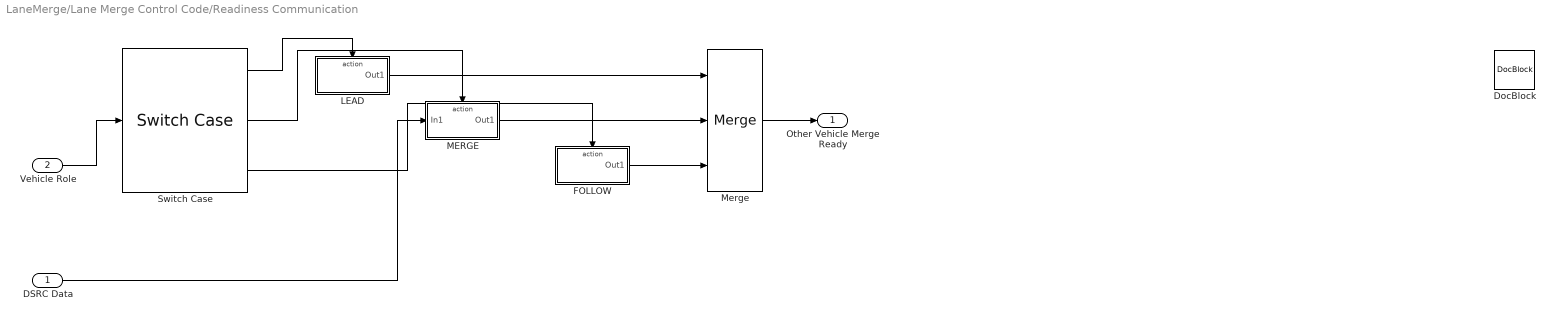
== system LaneMerge/Lane Merge Control Code/Readiness Communication ==
  DSRC Data : Inport  OutDataTypeStr=Bus: BSMStoreBus
  Vehicle Role : Inport  Port=2
  DocBlock : simulink/Model-Wide Utilities/DocBlock  DocumentType=Text
  FOLLOW : Subsystem  TreatAsAtomicUnit=on
  LEAD : Subsystem  TreatAsAtomicUnit=on
  MERGE : Subsystem  TreatAsAtomicUnit=on
  Merge : Merge  Inputs=3
  Switch Case : SwitchCase  CaseConditions={VehicleRoleEnum.LEAD, VehicleRoleEnum.MERGE, VehicleRoleEnum.FOLLOW}  ShowDefaultCase=off
  Other Vehicle Merge Ready : Outport
  wires:
  Switch Case/1 -> LEAD/Action
  Switch Case/2 -> MERGE/Action
  Switch Case/3 -> FOLLOW/Action
  Vehicle Role/1 -> Switch Case/1
  DSRC Data/1 -> MERGE/1(In1)
  FOLLOW/1(Out1) -> Merge/3
  MERGE/1(Out1) -> Merge/2
  LEAD/1(Out1) -> Merge/1
  Merge/1 -> Other Vehicle Merge Ready/1

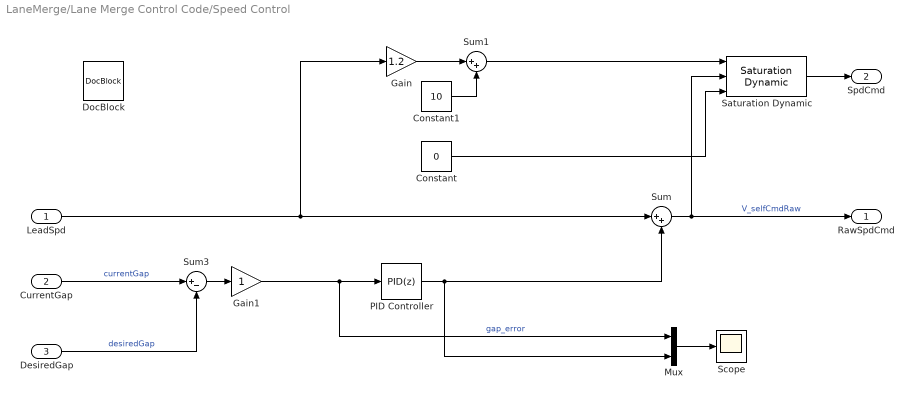
== system LaneMerge/Lane Merge Control Code/Speed Control ==
  LeadSpd : Inport
  CurrentGap : Inport  Port=2
  DesiredGap : Inport  Port=3
  Constant : Constant  Value=0
  Constant1 : Constant  Value=10
  DocBlock : simulink/Model-Wide Utilities/DocBlock  DocumentType=Text
      content=|
      | This block handles speed and gap control.
      |
      | This block attempts to minimize gap error via control of speed. It utilizes
      | a PID controller with gap error as the process variable and speed as the
      | manipulated variable. This PID outputs a speed command which is relative to
      | the lead vehicle's speed, thus it is added to the lead vehicle's speed to
      | get a desired speed value. Once the desired speed is computed it is run
      | through a saturation function to limit the values to between 0 and 1.2 *
      | Lead Vehicle Speed + 10.
  Gain : Gain  Gain=1.2
  Gain1 : Gain
  Mux : Mux  Inputs=2
  PID Controller : simulink/Continuous/PID Controller  Controller=PID  TimeDomain=Discrete-time  SampleTime=-1  IntegratorMethod=Forward Euler  FilterMethod=Forward Euler  Form=Parallel  P=0.75  I=0.01  D=0.15  N=10  InitialConditionSource=internal  InitialConditionForIntegrator=0  InitialConditionForFilter=0  ExternalReset=none  LimitOutput=on  UpperSaturationLimit=12  LowerSaturationLimit=-12  LinearizeAsGain=on  AntiWindupMode=back-calculation  Kb=1  TrackingMode=off  Kt=1  PParamMin=[]  PParamMax=[]  IParamMin=[]  IParamMax=[]  DParamMin=[]  DParamMax=[]  NParamMin=[]  NParamMax=[]  KbParamMin=[]  KbParamMax=[]  KtParamMin=[]  KtParamMax=[]  POutMin=[]  POutMax=[]  IOutMin=[]  IOutMax=[]  DOutMin=[]  DOutMax=[]  NOutMin=[]  NOutMax=[]  KbOutMin=[]  KbOutMax=[]  KtOutMin=[]  KtOutMax=[]  IntegratorOutMin=[]  IntegratorOutMax=[]  FilterOutMin=[]  FilterOutMax=[]  SumOutMin=[]  SumOutMax=[]  SumI1OutMin=[]  SumI1OutMax=[]  SumI2OutMin=[]  SumI2OutMax=[]  SumI3OutMin=[]  SumI3OutMax=[]  SumDOutMin=[]  SumDOutMax=[]  SaturationOutMin=[]  SaturationOutMax=[]  IntegratorContinuousStateAttributes=''  IntegratorStateMustResolveToSignalObject=off  IntegratorRTWStateStorageClass=Auto  FilterContinuousStateAttributes=''  FilterStateMustResolveToSignalObject=off  FilterRTWStateStorageClass=Auto
  Saturation Dynamic : simulink/Discontinuities/Saturation Dynamic  OutMin=[]  OutMax=[]  OutDataTypeStr=Inherit: Same as second input  OutDataType=fixdt(1, 16)  OutScaling=2^-10  DoSatur=off
  Scope : Scope
      settings: ShowLegends=on  YMin=-50  YMax=50  SaveName=ScopeData2  MaxDataPoints=15000
  Sum : Sum  Inputs=|++
  Sum1 : Sum  Inputs=|++
  Sum3 : Sum  Inputs=|+-
  RawSpdCmd : Outport
  SpdCmd : Outport  Port=2
  wires:
  Sum3/1 -> Gain1/1
  DesiredGap/1 -> Sum3/2  "desiredGap"
  Mux/1 -> Scope/1
  CurrentGap/1 -> Sum3/1  "currentGap"
  Sum/1 -> RawSpdCmd/1, Saturation Dynamic/2  "V_selfCmdRaw"
  Constant/1 -> Saturation Dynamic/3
  Sum1/1 -> Saturation Dynamic/1
  Gain/1 -> Sum1/1
  Constant1/1 -> Sum1/2
  Saturation Dynamic/1 -> SpdCmd/1
  PID Controller/1 -> Sum/2, Mux/2
  LeadSpd/1 -> Sum/1, Gain/1
  Gain1/1 -> PID Controller/1, Mux/1  "gap_error"

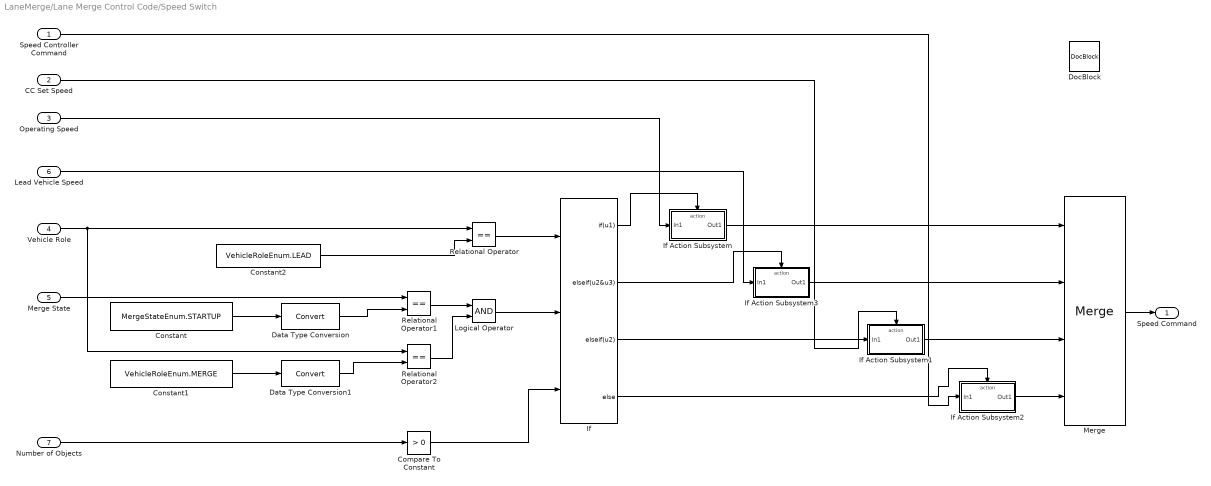
== system LaneMerge/Lane Merge Control Code/Speed Switch ==
  Speed Controller Command : Inport
  CC Set Speed : Inport  Port=2
  Operating Speed : Inport  Port=3
  Vehicle Role : Inport  Port=4
  Merge State : Inport  Port=5
  Lead Vehicle Speed : Inport  Port=6
  Number of Objects : Inport  Port=7
  Compare To Constant : simulink/Logic and Bit Operations/Compare To Constant  relop=>  const=0  OutDataTypeStr=boolean
  Constant : Constant  Value=MergeStateEnum.STARTUP
  Constant1 : Constant  Value=VehicleRoleEnum.MERGE
  Constant2 : Constant  Value=VehicleRoleEnum.LEAD
  Data Type Conversion : DataTypeConversion
  Data Type Conversion1 : DataTypeConversion
  DocBlock : simulink/Model-Wide Utilities/DocBlock  DocumentType=Text
  If : If  NumInputs=3  IfExpression=u1  ElseIfExpressions=u2&u3,u2
  If Action Subsystem : Subsystem  TreatAsAtomicUnit=on
  If Action Subsystem1 : Subsystem  TreatAsAtomicUnit=on
  If Action Subsystem2 : Subsystem  TreatAsAtomicUnit=on
  If Action Subsystem3 : Subsystem  TreatAsAtomicUnit=on
  Logical Operator : Logic  AllPortsSameDT=off  OutDataTypeStr=boolean
  Merge : Merge  Inputs=4
  Relational Operator : RelationalOperator  Operator===  OutDataTypeStr=boolean
  Relational Operator1 : RelationalOperator  Operator===  OutDataTypeStr=boolean
  Relational Operator2 : RelationalOperator  Operator===  OutDataTypeStr=boolean
  Speed Command : Outport
  wires:
  Vehicle Role/1 -> Relational Operator/1, Relational Operator2/1
  Constant2/1 -> Relational Operator/2
  Merge State/1 -> Relational Operator1/1
  Constant/1 -> Data Type Conversion/1
  Constant1/1 -> Data Type Conversion1/1
  Relational Operator2/1 -> Logical Operator/2
  Relational Operator1/1 -> Logical Operator/1
  Relational Operator/1 -> If/1
  Logical Operator/1 -> If/2
  If/1 -> If Action Subsystem/Action
  If/4 -> If Action Subsystem2/Action
  Speed Controller Command/1 -> If Action Subsystem2/1(In1)
  Operating Speed/1 -> If Action Subsystem/1(In1)
  CC Set Speed/1 -> If Action Subsystem1/1(In1)
  If Action Subsystem2/1(Out1) -> Merge/4
  If Action Subsystem1/1(Out1) -> Merge/3
  If Action Subsystem/1(Out1) -> Merge/1
  Merge/1 -> Speed Command/1
  Data Type Conversion/1 -> Relational Operator1/2
  Data Type Conversion1/1 -> Relational Operator2/2
  Number of Objects/1 -> Compare To Constant/1
  Compare To Constant/1 -> If/3
  If/3 -> If Action Subsystem1/Action
  If/2 -> If Action Subsystem3/Action
  Lead Vehicle Speed/1 -> If Action Subsystem3/1(In1)
  If Action Subsystem3/1(Out1) -> Merge/2

== system LaneMerge/RTI Data/RTI Data Store ==
  RTI Data Store : Subsystem  mask(RTI_DATA_STORE){}
      mask help:
      | RTI Data Store Block. This block is used by RTI to store internal model dependent data. Deleting this block will result in data loss.
      |
      | NEVER DELETE, COPY, OR MODIFY THIS BLOCK!
      mask Help:
      | RTI Data Store Block. This block is used by RTI to store internal model dependent data. Deleting this block will result in data loss.
      | 
      | NEVER DELETE, COPY, OR MODIFY THIS BLOCK!
      mask Display: text(0.5, 0.5, ' ', 'HorizontalAlignment', 'center');

== system LaneMerge/Lane Merge Control Code/CC Set Speed Latch/Latch Set ==
  In1 : Inport
  Trigger : TriggerPort
  Data Store Write : DataStoreWrite  DataStoreName=set_speed
  wires:
  In1/1 -> Data Store Write/1

== system LaneMerge/Lane Merge Control Code/Radar Target Speed/If Action Subsystem ==
  Relative Velocity : Inport
  CARMA Data : Inport  Port=2  OutDataTypeStr=Bus: GlobalStoreBus
  Action Port : ActionPort  ActionType=then
  Bus Selector : BusSelector  OutputSignals=speed_m_s.value
  Sum : Sum  Inputs=|++
  Lead Vehicle Speed : Outport
  wires:
  CARMA Data/1 -> Bus Selector/1
  Sum/1 -> Lead Vehicle Speed/1
  Bus Selector/1 -> Sum/2  "<value>"
  Relative Velocity/1 -> Sum/1

== system LaneMerge/Lane Merge Control Code/Radar Target Speed/If Action Subsystem1 ==
  Action Port : ActionPort  ActionType=else
  Constant : Constant  Value=0
  Out1 : Outport
  wires:
  Constant/1 -> Out1/1

== system LaneMerge/Lane Merge Control Code/Readiness Communication/FOLLOW ==
  Action Port : ActionPort  ActionType=case
  Constant : Constant  Value=true
  Out1 : Outport
  wires:
  Constant/1 -> Out1/1

== system LaneMerge/Lane Merge Control Code/Readiness Communication/LEAD ==
  Action Port : ActionPort  ActionType=case
  Constant : Constant  Value=true
  Out1 : Outport
  wires:
  Constant/1 -> Out1/1

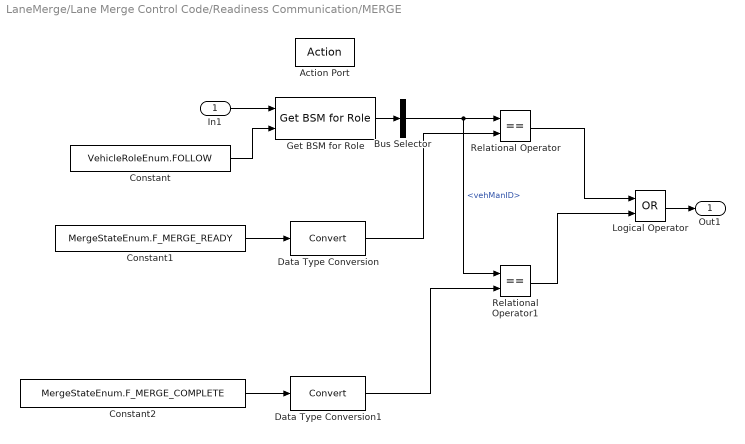
== system LaneMerge/Lane Merge Control Code/Readiness Communication/MERGE ==
  In1 : Inport
  Action Port : ActionPort  ActionType=case
  Bus Selector : BusSelector  OutputSignals=vehManID
  Constant : Constant  Value=VehicleRoleEnum.FOLLOW
  Constant1 : Constant  Value=MergeStateEnum.F_MERGE_READY
  Constant2 : Constant  Value=MergeStateEnum.F_MERGE_COMPLETE
  Data Type Conversion : DataTypeConversion
  Data Type Conversion1 : DataTypeConversion
  Get BSM for Role : dsrc_util_lib/Get BSM for Role
  Logical Operator : Logic  Operator=OR  AllPortsSameDT=off  OutDataTypeStr=boolean
  Relational Operator : RelationalOperator  Operator===  OutDataTypeStr=boolean
  Relational Operator1 : RelationalOperator  Operator===  OutDataTypeStr=boolean
  Out1 : Outport
  wires:
  In1/1 -> Get BSM for Role/1
  Constant/1 -> Get BSM for Role/2
  Get BSM for Role/1 -> Bus Selector/1
  Bus Selector/1 -> Relational Operator1/1, Relational Operator/1  "<vehManID>"
  Constant1/1 -> Data Type Conversion/1
  Relational Operator/1 -> Logical Operator/1
  Data Type Conversion/1 -> Relational Operator/2
  Constant2/1 -> Data Type Conversion1/1
  Data Type Conversion1/1 -> Relational Operator1/2
  Relational Operator1/1 -> Logical Operator/2
  Logical Operator/1 -> Out1/1

== system LaneMerge/Lane Merge Control Code/Speed Switch/If Action Subsystem ==
  In1 : Inport
  Action Port : ActionPort  ActionType=then
  Out1 : Outport
  wires:
  In1/1 -> Out1/1

== system LaneMerge/Lane Merge Control Code/Speed Switch/If Action Subsystem1 ==
  In1 : Inport
  Action Port : ActionPort  ActionType=elseif
  Out1 : Outport
  wires:
  In1/1 -> Out1/1

== system LaneMerge/Lane Merge Control Code/Speed Switch/If Action Subsystem2 ==
  In1 : Inport
  Action Port : ActionPort  ActionType=else
  Out1 : Outport
  wires:
  In1/1 -> Out1/1

== system LaneMerge/Lane Merge Control Code/Speed Switch/If Action Subsystem3 ==
  In1 : Inport
  Action Port : ActionPort  ActionType=elseif
  Out1 : Outport
  wires:
  In1/1 -> Out1/1

== system LaneMerge/RTI Data/RTI Data Store/RTI Data Store ==
  RTI Data Store : Subsystem  mask(RTI_DATA_STORE){}
      mask help:
      | RTI Data Store Block. This block is used by RTI to store internal model dependent data. Deleting this block will result in data loss.
      |
      | NEVER DELETE, COPY, OR MODIFY THIS BLOCK!
      mask Help:
      | RTI Data Store Block. This block is used by RTI to store internal model dependent data. Deleting this block will result in data loss.
      | 
      | NEVER DELETE, COPY, OR MODIFY THIS BLOCK!
      mask Display: text(0.5, 0.5, ' ', 'HorizontalAlignment', 'center');

== system LaneMerge/RTI Data/RTI Data Store/RTI Data Store/RTI Data Store ==
  RTI Data Store : Subsystem  mask(RTI_DATA_STORE){}
      mask help:
      | RTI Data Store Block. This block is used by RTI to store internal model dependent data. Deleting this block will result in data loss.
      |
      | NEVER DELETE, COPY, OR MODIFY THIS BLOCK!
      mask Help:
      | RTI Data Store Block. This block is used by RTI to store internal model dependent data. Deleting this block will result in data loss.
      | 
      | NEVER DELETE, COPY, OR MODIFY THIS BLOCK!
      mask Display: text(0.5, 0.5, ' ', 'HorizontalAlignment', 'center');

== system LaneMerge/RTI Data/RTI Data Store/RTI Data Store/RTI Data Store/RTI Data Store ==

== matlab function Lane Merge Control Code/Lightbar Controller/MATLAB Function ==
  data: state input double; lightbar output double
function lightbar = lights(state)
%#codegen

lightbar = [false, false, false, false];

if state == MergeStateEnum.MERGE_REQUEST
    lightbar(2) = true;
end

if state == MergeStateEnum.F_MERGE_REQUEST_ACK
    lightbar(1) = true;
end

if state == MergeStateEnum.M_MERGE_READY || state == MergeStateEnum.F_MERGE_READY
    lightbar(2) = true;
    lightbar(1) = true;
end

if state == MergeStateEnum.M_MERGE_COMPLETE || state == MergeStateEnum.F_MERGE_COMPLETE
    lightbar(3) = true;
    lightbar(2) = true;
    lightbar(1) = true;
end
